simulink model "A03_BoldMotSim"  (R2019a)
settings: Solver=VariableStepAuto  StartTime=0.0  StopTime=70  RelTol=1e-3
InitFcn:
  | A03_BoldMotSimVar
values from neighbouring files (symbols this model uses):
  setV_Norm = SamplesStepping.mVel    [A02_FreeMotSimVar.m]    (also in A03_BoldMotSimVar.m; Motor0_255_est.m = Samples(1:bfStart,3); MotorStepping.m = Samples(:,3); modelSimVar.m = Samples_10ms(1:bfStart,3))
  Ts = test.Time(2)    [A02_FreeMotSimVar.m]    (also in A03_BoldMotSimVar.m; Motor.m = floor(16000*1000*timeWanted/1024)*0.064*0.001; Motor0_255_est.m = floor(16000*1000*timeWanted/1024)*0.064*0.001; MotorMultipleCalc.m = floor(16000*1000*timeWanted/1024)*0.064*0.001)
  v0 = 0    [A02_FreeMotSimVar.m]    (also in A03_BoldMotSimVar.m; Motor0_255_est.m; MotorStepping.m; modelSimVar.m)
libraries: dspsrcs4 x3
settings Model: Creator=alfyhack  LastModifiedBy=alfyhack

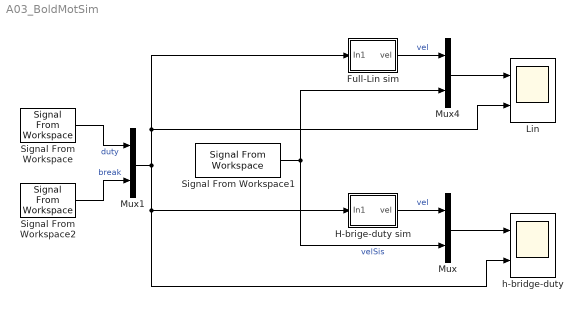
== system A03_BoldMotSim ==
  Full-Lin sim : Subsystem
  H-brige-duty sim : Subsystem
  Lin : Scope  NumInputPorts=2
  Mux : Mux  Inputs=2
  Mux1 : Mux  Inputs=2
  Mux4 : Mux  Inputs=2
  Signal From Workspace : dspsrcs4/Signal From Workspace  X=setU_Norm  Ts=Ts  nsamps=1  OutputAfterFinalValue=Setting to zero  ignoreOrWarnInputAndFrameLengths=off  OutputFrames=off
  Signal From Workspace1 : dspsrcs4/Signal From Workspace  X=[[0] [setV_Norm']]  Ts=Ts  nsamps=1  OutputAfterFinalValue=Setting to zero  ignoreOrWarnInputAndFrameLengths=off  OutputFrames=off
  Signal From Workspace2 : dspsrcs4/Signal From Workspace  X=setBrake  Ts=Ts  nsamps=1  OutputAfterFinalValue=Setting to zero  ignoreOrWarnInputAndFrameLengths=off  OutputFrames=off
  h-bridge-duty : Scope  NumInputPorts=2
  wires:
  Mux/1 -> h-bridge-duty/1
  Signal From Workspace2/1 -> Mux1/2  "break"
  Signal From Workspace/1 -> Mux1/1  "duty"
  H-brige-duty sim/1(vel) -> Mux/1  "vel"
  Full-Lin sim/1(vel) -> Mux4/1  "vel"
  Mux4/1 -> Lin/1
  Mux1/1 -> Full-Lin sim/1(In1), Lin/2, H-brige-duty sim/1(In1), h-bridge-duty/2
  Signal From Workspace1/1 -> Mux/2, Mux4/2  "velSis"

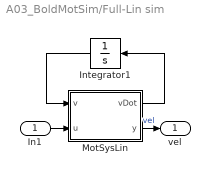
== system A03_BoldMotSim/Full-Lin sim ==
  In1 : Inport
  Integrator1 : Integrator  InitialCondition=v0
  MotSysLin : MATLAB Function  TreatAsAtomicUnit=on
  vel : Outport
  wires:
  Integrator1/1 -> MotSysLin/1(v)
  MotSysLin/1(vDot) -> Integrator1/1
  In1/1 -> MotSysLin/2(u)
  MotSysLin/2(y) -> vel/1  "vel"

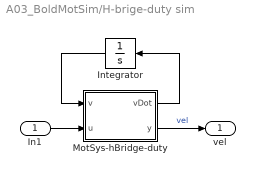
== system A03_BoldMotSim/H-brige-duty sim ==
  In1 : Inport
  Integrator : Integrator  InitialCondition=v0
  MotSys-hBridge-duty : MATLAB Function  TreatAsAtomicUnit=on
  vel : Outport
  wires:
  MotSys-hBridge-duty/1(vDot) -> Integrator/1
  In1/1 -> MotSys-hBridge-duty/2(u)
  Integrator/1 -> MotSys-hBridge-duty/1(v)
  MotSys-hBridge-duty/2(y) -> vel/1  "vel"

== matlab function A03_BoldMotSim/Full-Lin sim/MotSysLin ==
  data: v input; vDot output; u input; y output
function [vDot,y] = motor(v,u)
% u(1) = % pwm al motore
% u(2) = % Brake on/off

coder.extrinsic('evalin', 'assignin')

ka = 0;                  % Needed in order to set variable class correctly
ka = evalin('base','ka'); % Read value from workspace

rho = 0;                  % Needed in order to set variable class correctly
rho = evalin('base','rho'); % Read value from workspace


vDot = -rho*v + ka*u(1);

y=v;
end

== matlab function A03_BoldMotSim/H-brige-duty sim/MotSys-hBridge-duty ==
  data: v input; vDot output; u input; y output
function [vDot,y] = motor(v,u)
% u(1) = % pwm al motore
% u(2) = % Brake on/off

coder.extrinsic('evalin', 'assignin')

ka = 0;                  % Needed in order to set variable class correctly
ka = evalin('base','ka'); % Read value from workspace

rho = 0;                  % Needed in order to set variable class correctly
rho = evalin('base','rho'); % Read value from workspace

rhoMec = 0;                  % Needed in order to set variable class correctly
rhoMec = evalin('base','rhoMec'); % Read value from workspace

uDym = 0;
uDym = evalin('base','uDym'); % Read value from workspace

rhoInd = 0;                  % Needed in order to set variable class correctly
rhoInd = evalin('base','rhoInd'); % Read value from workspace

vDot=0;
if(~u(2))   % Non sono in frenata
    if(abs(v)>0.001)
        vDot = -((rhoInd)*abs(u(1)) + rhoMec + (uDym)/abs(v))*v + ka*u(1);
    else
        vDot = ka*u(1); % essendo fermo gli altri termini non ci sono
    end
else        % Sono in frenata
    if(abs(v)>0.001)
        vDot = -(rhoInd + rhoMec + (uDym)/abs(v))*v;
    end
end
y=v;
end
